simulink model "MQR_last_version"  (R2018a)
settings: Solver=FixedStepAuto  StartTime=0.0  StopTime=100  FixedStep=0.01  RelTol=1e-3
settings Model: Creator=icaro  LastModifiedBy=tarci

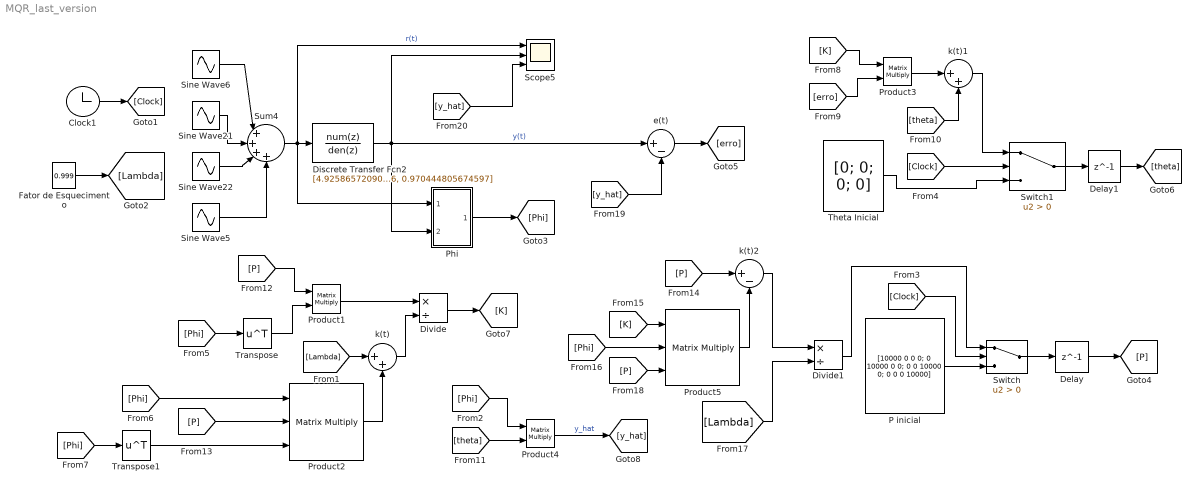
== system MQR_last_version ==
  Clock1 : Clock
  Delay : Delay  DelayLength=1  InitialCondition=0
  Delay1 : Delay  DelayLength=1  InitialCondition=0
  Discrete Transfer Fcn2 : DiscreteTransferFcn  Numerator=[4.92586572090045e-05, 9.85173144180090e-05, 4.92586572090045e-05]  Denominator=[1, -1.97024777104576, 0.970444805674597]
  Divide : Product  Inputs=*/
  Divide1 : Product  Inputs=*/
  "Fator de Esquecimento " : Constant  Value=0.999
  P inicial : Constant  Value=[10000 0 0 0; 0 10000 0 0; 0 0 10000 0; 0 0 0 10000]
  Phi : Subsystem
  Product1 : Product  Multiplication=Matrix(*)
  Product2 : Product  Inputs=3  Multiplication=Matrix(*)
  Product3 : Product  Multiplication=Matrix(*)
  Product4 : Product  Multiplication=Matrix(*)
  Product5 : Product  Inputs=3  Multiplication=Matrix(*)
  Scope5 : Scope  NumInputPorts=3
  Sine Wave21 : Sin  Frequency=0.2  SampleTime=0
  Sine Wave22 : Sin  Frequency=0.4  SampleTime=0
  Sine Wave5 : Sin  Frequency=0.8  SampleTime=0
  Sine Wave6 : Sin  Frequency=0.1  SampleTime=0
  Sum4 : Sum  Inputs=|++++
  Switch : Switch  Criteria=u2 > Threshold
  Switch1 : Switch  Criteria=u2 > Threshold
  "Theta Inicial " : Constant  Value=[0; 0; 0; 0]
  Transpose : Math  Operator=transpose  SaturateOnIntegerOverflow=on
  Transpose1 : Math  Operator=transpose  SaturateOnIntegerOverflow=on
  e(t) : Sum  Inputs=|+-
  k(t) : Sum  Inputs=|++
  k(t)1 : Sum  Inputs=|++
  k(t)2 : Sum  Inputs=|+-
  wires:
  Discrete Transfer Fcn2/1 -> e(t)/1, Scope5/2, Phi/2(y(t))  "y(t)"
  Sine Wave6/1 -> Sum4/1
  Sine Wave21/1 -> Sum4/2
  Sine Wave22/1 -> Sum4/3
  Sine Wave5/1 -> Sum4/4
  Sum4/1 -> Discrete Transfer Fcn2/1, Phi/1(r(t)), Scope5/1  "r(t)"
  "Theta Inicial "/1 -> Switch1/3
  [Clock] -> Switch1/2
  Clock1/1 -> [Clock]
  e(t)/1 -> [erro]
  [Clock] -> Switch/2
  P inicial/1 -> Switch/3
  [P] -> Product1/1
  Transpose/1 -> Product1/2
  Product1/1 -> Divide/1
  "Fator de Esquecimento "/1 -> [Lambda]
  [Lambda] -> k(t)/1
  Phi/1(Phi) -> [Phi]
  [Phi] -> Transpose/1
  Product2/1 -> k(t)/2
  [Phi] -> Product2/1
  [Phi] -> Transpose1/1
  Transpose1/1 -> Product2/3
  Switch1/1 -> Delay1/1
  [K] -> Product3/1
  [erro] -> Product3/2
  Product3/1 -> k(t)1/1
  [theta] -> k(t)1/2
  k(t)1/1 -> Switch1/1
  Divide/1 -> [K]
  [P] -> Product2/2
  k(t)/1 -> Divide/2
  [P] -> k(t)2/1
  [K] -> Product5/1
  [Phi] -> Product5/2
  [Lambda] -> Divide1/2
  [P] -> Product5/3
  Switch/1 -> Delay/1
  Divide1/1 -> Switch/1
  Product5/1 -> k(t)2/2
  k(t)2/1 -> Divide1/1
  [theta] -> Product4/2
  [Phi] -> Product4/1
  Product4/1 -> [y_hat]  "y_hat"
  [y_hat] -> e(t)/2
  [y_hat] -> Scope5/3
  Delay/1 -> [P]
  Delay1/1 -> [theta]

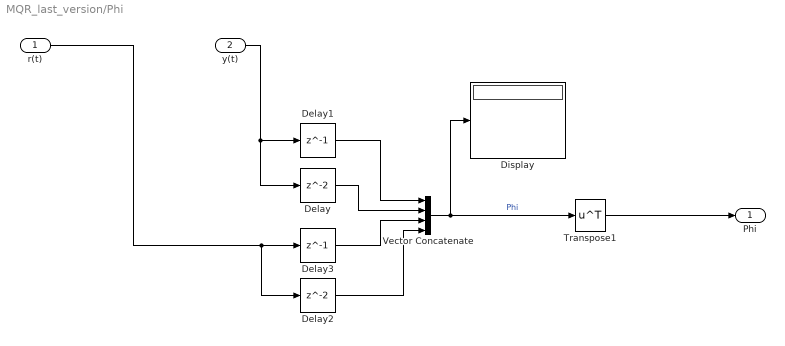
== system MQR_last_version/Phi ==
  r(t) : Inport
  y(t) : Inport  Port=2
  Delay : Delay
  Delay1 : Delay  DelayLength=1
  Delay2 : Delay
  Delay3 : Delay  DelayLength=1
  Display : Display
  Transpose1 : Math  Operator=transpose  SaturateOnIntegerOverflow=on
  Vector Concatenate : Concatenate  NumInputs=4
  Phi : Outport
  wires:
  r(t)/1 -> Delay2/1, Delay3/1
  Vector Concatenate/1 -> Transpose1/1, Display/1  "Phi"
  Delay/1 -> Vector Concatenate/2
  y(t)/1 -> Delay/1, Delay1/1
  Delay3/1 -> Vector Concatenate/3
  Delay2/1 -> Vector Concatenate/4
  Delay1/1 -> Vector Concatenate/1
  Transpose1/1 -> Phi/1
